simulink model "four_link_model"  (R2022a)
settings: Solver=VariableStepAuto  StartTime=0.0  StopTime=10.0  RelTol=1e-3
settings Model: Creator=org  LastModifiedBy=org

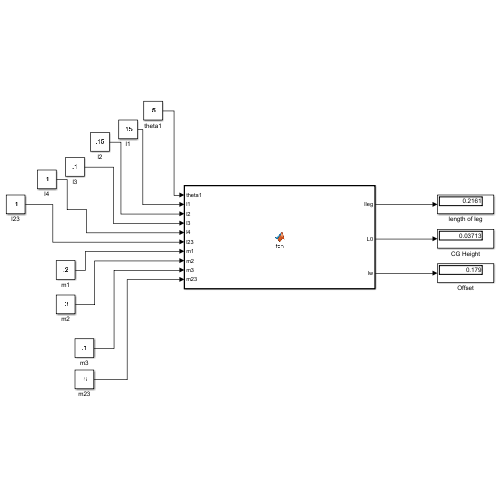
[thumbnail: Simulink's stored preview of the top-level diagram]
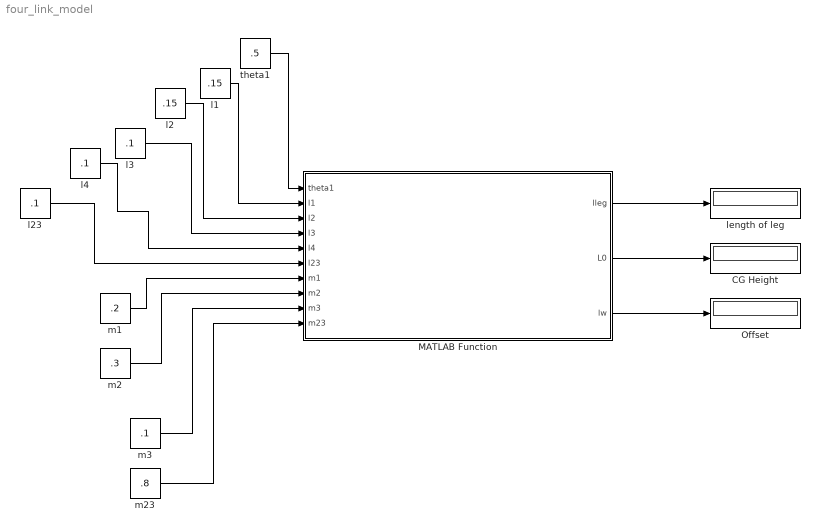
== system four_link_model ==
  CG Height : Display
  MATLAB Function : MATLAB Function  TreatAsAtomicUnit=on
  Offset : Display
  l1 : Constant  Value=.15
  l2 : Constant  Value=.15
  l23 : Constant  Value=.1
  l3 : Constant  Value=.1
  l4 : Constant  Value=.1
  length of leg : Display
  m1 : Constant  Value=.2
  m2 : Constant  Value=.3
  m23 : Constant  Value=.8
  m3 : Constant  Value=.1
  theta1 : Constant  Value=.5
  wires:
  theta1/1 -> MATLAB Function/1(theta1)
  l1/1 -> MATLAB Function/2(l1)
  l2/1 -> MATLAB Function/3(l2)
  l3/1 -> MATLAB Function/4(l3)
  l4/1 -> MATLAB Function/5(l4)
  l23/1 -> MATLAB Function/6(l23)
  m1/1 -> MATLAB Function/7(m1)
  m2/1 -> MATLAB Function/8(m2)
  m3/1 -> MATLAB Function/9(m3)
  m23/1 -> MATLAB Function/10(m23)
  MATLAB Function/1(lleg) -> length of leg/1
  MATLAB Function/2(L0) -> CG Height/1
  MATLAB Function/3(lw) -> Offset/1

== matlab function four_link_model/MATLAB Function ==
  data: theta1 input; l1 input; l2 input; l3 input; l4 input; l23 input; m1 input; m2 input; m3 input; m23 input; lleg output; L0 output; lw output
function [lleg, L0, lw] = fcn(theta1, l1, l2, l3, l4, l23, m1, m2, m3, m23)
    
    
    l5 = sqrt(l2^2 + l4^2 - 2 * l2 * l4 * cos(theta1 + pi/4));
    theta2 = asin((l4 * sin(theta1 + pi/4)) / l5);
    theta3 = acos((l23^2 + l5^2 - l3^2) / (2 * l23 * l5));
    theta4 = pi - theta1 - theta2 - theta3;
    theta5 = pi - theta4;
    theta6 = asin((l5 * sin(theta3)) / l3) - theta4;
    

    lleg = l2 * sin(theta1) + l1 * sin(theta4);
    
   
    xc2 = (l2 * sin(theta1)) / 2;
    xc1 = l2 * sin(theta1) + (l1 * sin(theta5)) / 2;
    xc3 = -l4 * sin(pi/4) + (l3 * sin(theta6)) / 2;
    xc23 = l2 * sin(theta1) - (l23 * sin(theta4)) / 2;
    

    L0 = (m1*xc1 + m2*xc2 + m3*xc3 + m23*xc23) / (m1 + m2 + m3 + m23);
    
   
    lw = lleg - L0;
    
end
